simulink model "lv_tansfer"  (Simulink 7.1)
settings: Solver=ode45  StartTime=0.0  StopTime=100  RelTol=1e-3
values from neighbouring files (symbols this model uses):
  Jem = 90    [lv_cankaofile.m]    (also in lv_demofile.m = 97.5; lv_demofile1.m = 97.5; lv_demofile2.m = 97.5; lv_demofile3.m = 97.5)
  Jwt = 9e7    (= 90000000)    [lv_cankaofile.m]    (also in lv_demofile.m = 3275300; lv_demofile1.m = 3275300; lv_demofile2.m = 3275300; lv_demofile3.m = 3275300)
  K = 83    [lv_cankaofile.m]    (also in lv_demofile.m; lv_demofile1.m = 75.76; lv_demofile2.m; lv_demofile3.m = 75.76)
settings Model: Creator=lv  LastModifiedBy=lv

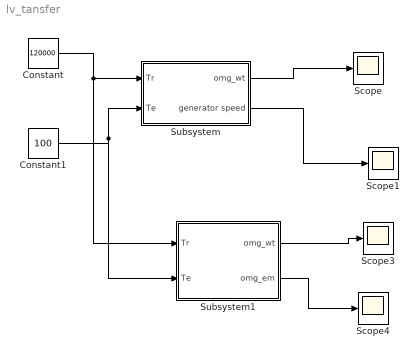
== system lv_tansfer ==
  Constant : Constant  Value=120000  OutDataType=sfix(16)  OutScaling=2^0
  Constant1 : Constant  Value=100  OutDataType=sfix(16)  OutScaling=2^0
  Scope{,1,3..4} (4 alike) : Scope
      Scope3 settings: SaveName=ScopeData3
      Scope4 settings: SaveName=ScopeData4
  Subsystem : Subsystem
  Subsystem1 : Subsystem
  wires:
  Constant/1 -> Subsystem/1(Tr), Subsystem1/1(Tr)
  Constant1/1 -> Subsystem/2(Te), Subsystem1/2(Te)
  Subsystem/1(omg_wt) -> Scope/1
  Subsystem/2(generator speed) -> Scope1/1
  Subsystem1/1(omg_wt) -> Scope3/1
  Subsystem1/2(omg_em) -> Scope4/1

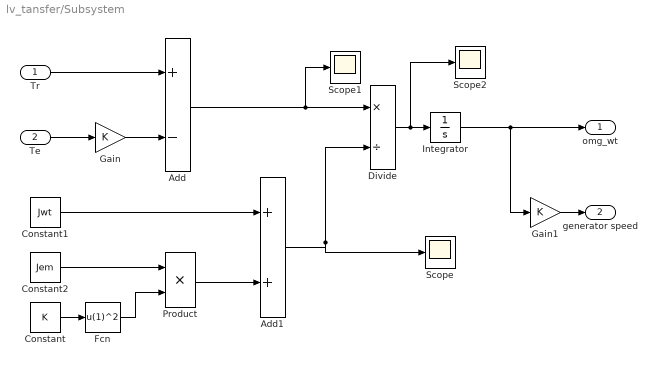
== system lv_tansfer/Subsystem ==
  Tr : Inport  OutDataType=sfix(16)  OutScaling=2^0
  Te : Inport  Port=2  OutDataType=sfix(16)  OutScaling=2^0
  Add : Sum  Inputs=+-  OutDataType=sfix(16)  OutScaling=2^-10
  Add1 : Sum  OutDataType=sfix(16)  OutScaling=2^-10
  Constant : Constant  Value=K  OutDataType=sfix(16)  OutScaling=2^0
  Constant1 : Constant  Value=Jwt  OutDataType=sfix(16)  OutScaling=2^0
  Constant2 : Constant  Value=Jem  OutDataType=sfix(16)  OutScaling=2^0
  Divide : Product  Inputs=*/  OutDataType=sfix(16)  OutScaling=2^-10
  Fcn : Fcn  Expr=u(1)^2
  Gain : Gain  Gain=K  ParameterDataType=sfix(16)  ParameterScaling=2^0  OutDataType=sfix(16)  OutScaling=2^0
  Gain1 : Gain  Gain=K  ParameterDataType=sfix(16)  ParameterScaling=2^0  OutDataType=sfix(16)  OutScaling=2^0
  Integrator : Integrator
  Product : Product  OutDataType=sfix(16)  OutScaling=2^0  RndMeth=Zero
  Scope : Scope
      settings: SaveName=ScopeData5
  Scope1 : Scope
      settings: SaveName=ScopeData6
  Scope2 : Scope
      settings: SaveName=ScopeData7
  omg_wt : Outport  OutDataType=sfix(16)  OutScaling=2^0
  generator speed : Outport  Port=2  OutDataType=sfix(16)  OutScaling=2^0
  wires:
  Gain1/1 -> generator speed/1
  Integrator/1 -> omg_wt/1, Gain1/1
  Divide/1 -> Integrator/1, Scope2/1
  Add1/1 -> Divide/2, Scope/1
  Add/1 -> Divide/1, Scope1/1
  Product/1 -> Add1/2
  Constant1/1 -> Add1/1
  Constant2/1 -> Product/1
  Gain/1 -> Add/2
  Tr/1 -> Add/1
  Te/1 -> Gain/1
  Constant/1 -> Fcn/1
  Fcn/1 -> Product/2

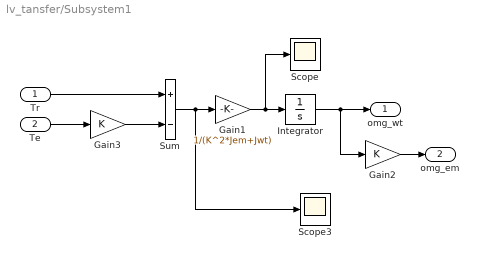
== system lv_tansfer/Subsystem1 ==
  Tr : Inport  OutDataType=sfix(16)  OutScaling=2^0
  Te : Inport  Port=2  OutDataType=sfix(16)  OutScaling=2^0
  Gain1 : Gain  Gain=1/(K^2*Jem+Jwt)  ParameterDataType=sfix(16)  ParameterScaling=2^0  OutDataType=sfix(16)  OutScaling=2^0  SaturateOnIntegerOverflow=on  OutDataTypeStr=Inherit: Same as input  ParamDataTypeStr=Inherit: Same as input
  Gain2 : Gain  Gain=K  ParameterDataType=sfix(16)  ParameterScaling=2^0  OutDataType=sfix(16)  OutScaling=2^0  SaturateOnIntegerOverflow=on  OutDataTypeStr=Inherit: Same as input  ParamDataTypeStr=Inherit: Same as input
  Gain3 : Gain  Gain=K  ParameterDataType=sfix(16)  ParameterScaling=2^0  OutDataType=sfix(16)  OutScaling=2^0  SaturateOnIntegerOverflow=on  OutDataTypeStr=Inherit: Same as input  ParamDataTypeStr=Inherit: Same as input
  Integrator : Integrator
  Scope : Scope
      settings: SaveName=ScopeData8
  Scope3 : Scope
      settings: SaveName=ScopeData2
  Sum : Sum  Inputs=+-  OutDataType=sfix(16)  OutScaling=2^0  SaturateOnIntegerOverflow=on  InputSameDT=on  OutDataTypeStr=Inherit: Same as first input
  omg_wt : Outport  OutDataType=sfix(16)  OutScaling=2^0  InitialOutput=0
  omg_em : Outport  Port=2  OutDataType=sfix(16)  OutScaling=2^0  InitialOutput=0
  wires:
  Gain1/1 -> Scope/1, Integrator/1
  Sum/1 -> Gain1/1, Scope3/1
  Te/1 -> Gain3/1
  Tr/1 -> Sum/1
  Gain2/1 -> omg_em/1
  Gain3/1 -> Sum/2
  Integrator/1 -> omg_wt/1, Gain2/1
